simulink model "GT_hover"  (R2024a)
settings: Solver=ode4  StartTime=0.0  StopTime=5  FixedStep=1/1600  RelTol=1e-3
undefined symbols (not defined in the file): Earth, H0, result_hover, WGS84, wind_x, wind_y, wind_z
libraries: Sensors x3, PosControl x1, GT x1, aerolibtransform2 x1, aerolibnav x1
settings Model: Creator=igmso  LastModifiedBy=igmso
settings DataIOCC: ExternalInput=[t,u]  InitialState=getstatestruct(op_trim3)  SaveFormat=StructureWithTime

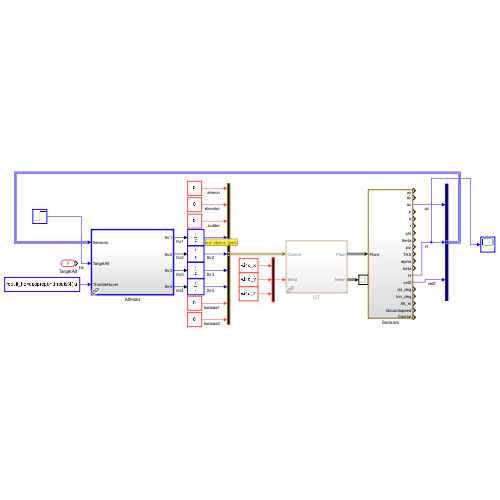
[thumbnail: Simulink's stored preview of the top-level diagram]
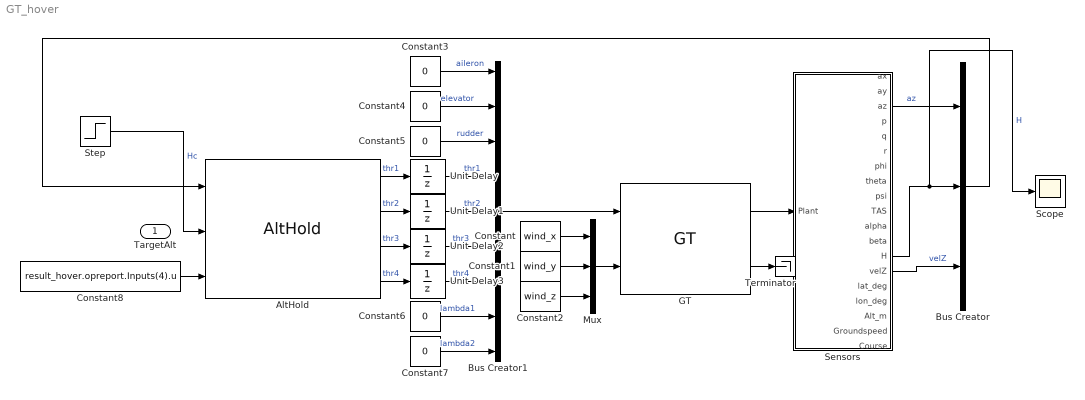
== system GT_hover ==
  TargetAlt : Inport
  AltHold : PosControl/AltHold  SystemSampleTime=-1  VariantActivationTime=update diagram  AllowFlexibleInterface=on  Latency=0  AutoFrameSizeCalculation=off
  Bus Creator1 : BusCreator  Inputs=9
  Bus Creator : BusCreator  Inputs=3
  Constant : Constant  Value=wind_x  SampleTime=-1
  Constant1 : Constant  Value=wind_y  SampleTime=-1
  Constant2 : Constant  Value=wind_z  SampleTime=-1
  Constant{3..7} (5 alike) : Constant  Value=0  SampleTime=-1
  Constant8 : Constant  Value=result_hover.opreport.Inputs(4).u  SampleTime=-1
  GT : GT/GT  SystemSampleTime=-1  VariantActivationTime=update diagram  AllowFlexibleInterface=on  Latency=0  AutoFrameSizeCalculation=off
  Mux : Mux  Inputs=3
  Scope : Scope
  Sensors : Subsystem
  Step : Step  Time=5  Before=H0  After=H0+30
  Terminator : Terminator
  Unit Delay{,1..3} (4 alike) : UnitDelay  SampleTime=-1  HasFrameUpgradeWarning=on
  wires:
  Constant8/1 -> AltHold/3
  Step/1 -> AltHold/2  "Hc"
  AltHold/4 -> Unit Delay3/1  "thr4"
  AltHold/3 -> Unit Delay2/1  "thr3"
  AltHold/1 -> Unit Delay/1  "thr1"
  AltHold/2 -> Unit Delay1/1  "thr2"
  Mux/1 -> GT/2
  GT/2 -> Terminator/1
  Bus Creator1/1 -> GT/1
  Constant2/1 -> Mux/3
  GT/1 -> Sensors/1(Plant)
  Constant5/1 -> Bus Creator1/3  "rudder"
  Constant3/1 -> Bus Creator1/1  "aileron"
  Constant7/1 -> Bus Creator1/9  "lambda2"
  Constant4/1 -> Bus Creator1/2  "elevator"
  Constant/1 -> Mux/1
  Constant1/1 -> Mux/2
  Constant6/1 -> Bus Creator1/8  "lambda1"
  Sensors/3(az) -> Bus Creator/1  "az"
  Sensors/13(H) -> Scope/1, Bus Creator/2  "H"
  Sensors/14(velZ) -> Bus Creator/3  "velZ"
  Bus Creator/1 -> AltHold/1
  Unit Delay/1 -> Bus Creator1/4  "thr1"
  Unit Delay1/1 -> Bus Creator1/5  "thr2"
  Unit Delay2/1 -> Bus Creator1/6  "thr3"
  Unit Delay3/1 -> Bus Creator1/7  "thr4"

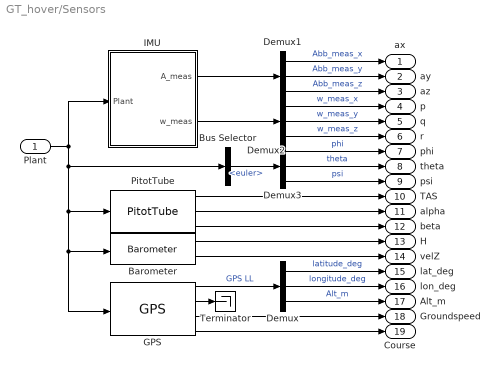
== system GT_hover/Sensors ==
  Plant : Inport
  Barometer : Sensors/Barometer  SystemSampleTime=1/400  VariantActivationTime=update diagram  AllowFlexibleInterface=on  Latency=0  AutoFrameSizeCalculation=off
  Bus Selector : BusSelector  OutputSignals=euler
  Demux{,1..3} (4 alike) : Demux  Outputs=3
  GPS : Sensors/GPS  SystemSampleTime=1/400  VariantActivationTime=update diagram  AllowFlexibleInterface=on  Latency=0  AutoFrameSizeCalculation=off
  IMU : Subsystem  AncestorBlock=Sensors/IMU  TreatAsAtomicUnit=on
  PitotTube : Sensors/PitotTube  SystemSampleTime=1/400  VariantActivationTime=update diagram  AllowFlexibleInterface=on  Latency=0  AutoFrameSizeCalculation=off
  Terminator : Terminator
  ax : Outport
  ay : Outport  Port=2
  az : Outport  Port=3
  p : Outport  Port=4
  q : Outport  Port=5
  r : Outport  Port=6
  phi : Outport  Port=7
  theta : Outport  Port=8
  psi : Outport  Port=9
  TAS : Outport  Port=10
  alpha : Outport  Port=11
  beta : Outport  Port=12
  H : Outport  Port=13
  velZ : Outport  Port=14
  lat_deg : Outport  Port=15
  lon_deg : Outport  Port=16
  Alt_m : Outport  Port=17
  Groundspeed : Outport  Port=18
  Course : Outport  Port=19
  wires:
  Barometer/1 -> H/1
  GPS/2 -> Terminator/1
  GPS/3 -> Groundspeed/1
  GPS/4 -> Course/1
  Plant/1 -> GPS/1, Barometer/1, PitotTube/1, Bus Selector/1, IMU/1(Plant)
  Demux/1 -> lat_deg/1  "latitude_deg"
  Demux/2 -> lon_deg/1  "longitude_deg"
  Demux/3 -> Alt_m/1  "Alt_m"
  PitotTube/1 -> TAS/1
  PitotTube/2 -> alpha/1
  PitotTube/3 -> beta/1
  Demux1/3 -> az/1  "Abb_meas_z"
  Demux1/2 -> ay/1  "Abb_meas_y"
  Demux1/1 -> ax/1  "Abb_meas_x"
  IMU/1(A_meas) -> Demux1/1
  IMU/2(w_meas) -> Demux2/1
  Demux2/1 -> p/1  "w_meas_x"
  Demux2/2 -> q/1  "w_meas_y"
  Demux2/3 -> r/1  "w_meas_z"
  Barometer/2 -> velZ/1
  GPS/1 -> Demux/1  "GPS LL"
  Bus Selector/1 -> Demux3/1  "<euler>"
  Demux3/1 -> phi/1  "phi"
  Demux3/2 -> theta/1  "theta"
  Demux3/3 -> psi/1  "psi"

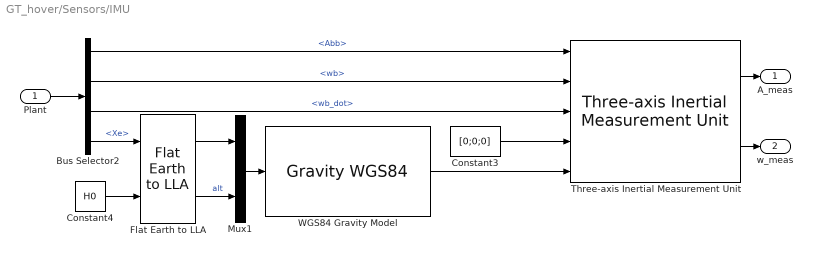
== system GT_hover/Sensors/IMU ==
  Plant : Inport  SampleTime=1/400
  Bus Selector2 : BusSelector  OutputSignals=Abb,wb,wb_dot,Xe
  Constant3 : Constant  Value=[0;0;0]  SampleTime=-1
  Constant4 : Constant  Value=H0  SampleTime=-1
  Flat Earth to LLA : aerolibtransform2/Flat Earth to LLA  units=Metric (MKS)  ptype=Earth (WGS84)  F=1/298.257223563  R=6378137  refPosPort=off  LL0=SJK_airport  psi=SJK_direction
  Mux1 : Mux  Inputs=2
  Three-axis Inertial Measurement Unit : aerolibnav/Three-axis Inertial Measurement Unit  units=Metric (MKS)  imu=[0 0 0]  i_Ts=1/800  dtype_a=on  w_a=190  z_a=0.707  a_sf_cc=[1 0 0; 0 1 0; 0 0 1]  a_bias=[0 0 0]  a_sat="[-inf  -inf  -inf  inf inf inf]"  dtype_g=on  w_g=190  z_g=0.707  g_sf_cc=[1 0 0; 0 1 0; 0 0 1]  g_bias=[0 0 0]  g_sens=[0 0 0]  g_sat="[-inf  -inf  -inf  inf inf inf]"  i_rand=on  i_seeds=[23093 23094 23095 23096 23097 23098]  i_pow=[0.001 0.001 0.001 0.0001 0.0001 0.0001]
  "WGS84 Gravity Model  " : GravityWGS84
  A_meas : Outport  SampleTime=1/400
  w_meas : Outport  Port=2  SampleTime=1/400
  wires:
  Bus Selector2/2 -> Three-axis Inertial Measurement Unit/2  "<wb>"
  Constant3/1 -> Three-axis Inertial Measurement Unit/4
  Bus Selector2/3 -> Three-axis Inertial Measurement Unit/3  "<wb_dot>"
  Mux1/1 -> "WGS84 Gravity Model  "/1
  Plant/1 -> Bus Selector2/1
  Bus Selector2/4 -> Flat Earth to LLA/1  "<Xe>"
  "WGS84 Gravity Model  "/1 -> Three-axis Inertial Measurement Unit/5
  Bus Selector2/1 -> Three-axis Inertial Measurement Unit/1  "<Abb>"
  Flat Earth to LLA/2 -> Mux1/2  "alt"
  Constant4/1 -> Flat Earth to LLA/2
  Flat Earth to LLA/1 -> Mux1/1
  Three-axis Inertial Measurement Unit/2 -> w_meas/1
  Three-axis Inertial Measurement Unit/1 -> A_meas/1
